simulink model "sistema_velocidad"  (R2014b)
settings: Solver=ode4  SolverMode=SingleTasking  StartTime=0.0  StopTime=tfin+ts  FixedStep=ts  MaxStep=ts  RelTol=1e-6  AbsTol=1e-9
values from neighbouring files (symbols this model uses):
  ts = 0.005    [ControlP.m]    (also in ControlPID_RF.m; DatosIdentVel_rampa.mat)
undefined symbols (not defined in the file or in its folder): th
settings Model: ExtModeTrigMode=oneshot  ExtModeArmWhenConnect=off  BufferReuse=off  Creator=zamora  LastModifiedBy=zamora
settings SolverCC: ZeroCrossAlgorithm=Adaptive
settings DataIOCC: LimitDataPoints=off  SignalLoggingSaveFormat=ModelDataLogs  SaveOutput=off  SaveTime=off  StateSaveName=x  TimeSaveName=t  OutputSaveName=y
settings OptimizationCC: BlockReduction=off  BooleanDataType=off  InlineParams=on  BufferReuse=off  ExpressionDepthLimit=2147483647
settings DebuggingCC: SaveWithParameterizedLinksMsg=none  UnderspecifiedInitializationDetection=Classic  MergeDetectMultiDrivingBlocksExec=none  SignalResolutionControl=TryResolveAllWithWarning  MaxConsecutiveZCsMsg=none  IgnoredZcDiagnostic=none  SolverPrmCheckMsg=none  MultiTaskDSMMsg=warning  MultiTaskCondExecSysMsg=none  FcnCallInpInsideContextMsg=EnableAllAsWarning  StateNameClashWarn=warning
settings HardwareCC: TargetUnknown=on
settings RTWCC: TemplateMakefile=grt_unix.tmf  IncludeERTFirstTime=on
settings GRTTargetCC: CombineOutputUpdateFcns=off  GRTInterface=on

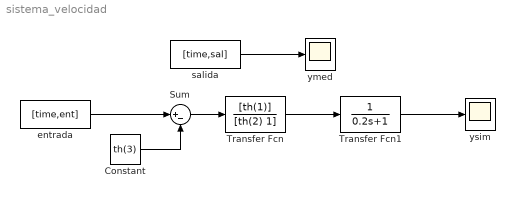
== system sistema_velocidad ==
  Constant : Constant  Value=th(3)  SampleTime=0
  Sum : Sum  Inputs=|+-
  Transfer Fcn : TransferFcn  Numerator=[th(1)]  Denominator=[th(2) 1]
  Transfer Fcn1 : TransferFcn  Numerator=1  Denominator=[0.2 1]
  entrada : FromWorkspace  VariableName=[time,ent]  SampleTime=ts
  salida : FromWorkspace  VariableName=[time,sal]  SampleTime=ts
  ymed : Scope
      settings: SaveName=ymed  SampleInput=on  SampleTime=ts
  ysim : Scope
      settings: SaveName=ysim  SampleInput=on  SampleTime=ts
  wires:
  salida/1 -> ymed/1
  Transfer Fcn1/1 -> ysim/1
  Transfer Fcn/1 -> Transfer Fcn1/1
  entrada/1 -> Sum/1
  Sum/1 -> Transfer Fcn/1
  Constant/1 -> Sum/2
